simulink subsystem "packs_temperatures_12"  (R2020b)
settings: Solver=VariableStepAuto  StartTime=0.0  StopTime=10.0  RelTol=1e-3
undefined symbols (not defined in the file): bufferSize, params_packs_temperatures_12, possible_ppms
libraries: cstblocks x12
settings Model: Creator=leop9  LastModifiedBy=Previ

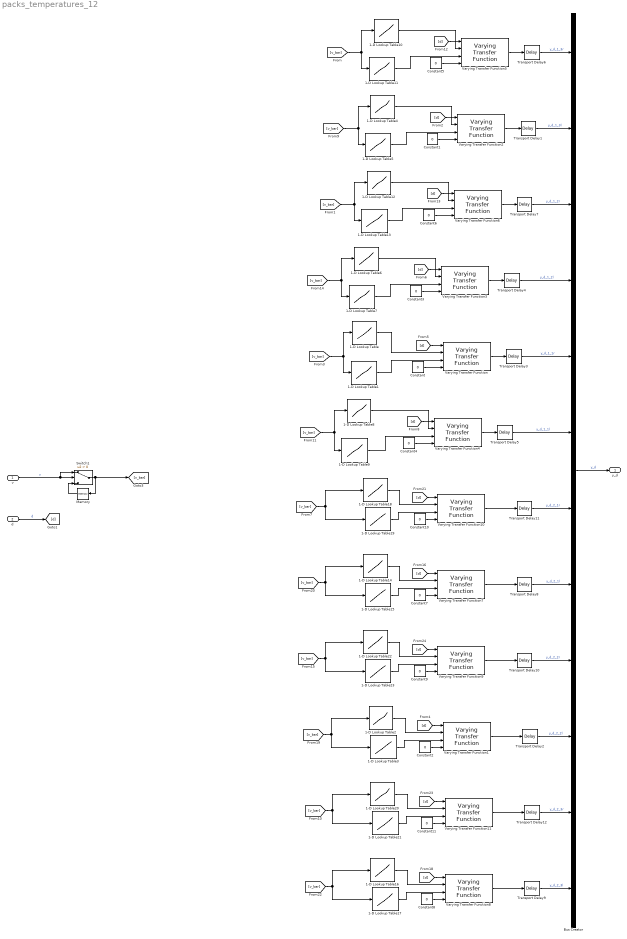
== system packs_temperatures_12 ==
  v : Inport
  d : Inport  Port=2
  1-D Lookup Table : Lookup_n-D  NumberOfTableDimensions=1  BreakpointsForDimension1=possible_ppms  BreakpointsForDimension2=[0,30,60,90]  Table=[params_packs_temperatures_12.T1_1r.b0(1),params_packs_temperatures_12.T1_1r.b0(2),params_packs_temperatures_12.T1_1r.b0(3)]  InternalRulePriority=Speed  RndMeth=Simplest  InputSameDT=on
  1-D Lookup Table1 : Lookup_n-D  NumberOfTableDimensions=1  BreakpointsForDimension1=possible_ppms  BreakpointsForDimension2=[0,30,60,90]  Table=[params_packs_temperatures_12.T1_1r.a0(1),params_packs_temperatures_12.T1_1r.a0(2),params_packs_temperatures_12.T1_1r.a0(3)]  InternalRulePriority=Speed  RndMeth=Simplest  InputSameDT=on
  1-D Lookup Table10 : Lookup_n-D  NumberOfTableDimensions=1  BreakpointsForDimension1=possible_ppms  BreakpointsForDimension2=[0,30,60,90]  Table=[params_packs_temperatures_12.T1_3r.b0(1),params_packs_temperatures_12.T1_3r.b0(2),params_packs_temperatures_12.T1_3r.b0(3)]  InternalRulePriority=Speed  RndMeth=Simplest  InputSameDT=on
  1-D Lookup Table11 : Lookup_n-D  NumberOfTableDimensions=1  BreakpointsForDimension1=possible_ppms  BreakpointsForDimension2=[0,30,60,90]  Table=[params_packs_temperatures_12.T1_3r.a0(1),params_packs_temperatures_12.T1_3r.a0(2),params_packs_temperatures_12.T1_3r.a0(3)]  InternalRulePriority=Speed  RndMeth=Simplest  InputSameDT=on
  1-D Lookup Table12 : Lookup_n-D  NumberOfTableDimensions=1  BreakpointsForDimension1=possible_ppms  BreakpointsForDimension2=[0,30,60,90]  Table=[params_packs_temperatures_12.T1_2r.b0(1),params_packs_temperatures_12.T1_2r.b0(2),params_packs_temperatures_12.T1_2r.b0(3)]  InternalRulePriority=Speed  RndMeth=Simplest  InputSameDT=on
  1-D Lookup Table13 : Lookup_n-D  NumberOfTableDimensions=1  BreakpointsForDimension1=possible_ppms  BreakpointsForDimension2=[0,30,60,90]  Table=[params_packs_temperatures_12.T1_2r.a0(1),params_packs_temperatures_12.T1_2r.a0(2),params_packs_temperatures_12.T1_2r.a0(3)]  InternalRulePriority=Speed  RndMeth=Simplest  InputSameDT=on
  1-D Lookup Table14 : Lookup_n-D  NumberOfTableDimensions=1  BreakpointsForDimension1=possible_ppms  BreakpointsForDimension2=[0,30,60,90]  Table=[params_packs_temperatures_12.T2_1l.b0(1),params_packs_temperatures_12.T2_1l.b0(2),params_packs_temperatures_12.T2_1l.b0(3)]  InternalRulePriority=Speed  RndMeth=Simplest  InputSameDT=on
  1-D Lookup Table15 : Lookup_n-D  NumberOfTableDimensions=1  BreakpointsForDimension1=possible_ppms  BreakpointsForDimension2=[0,30,60,90]  Table=[params_packs_temperatures_12.T2_1l.a0(1),params_packs_temperatures_12.T2_1l.a0(2),params_packs_temperatures_12.T2_1l.a0(3)]  InternalRulePriority=Speed  RndMeth=Simplest  InputSameDT=on
  1-D Lookup Table16 : Lookup_n-D  NumberOfTableDimensions=1  BreakpointsForDimension1=possible_ppms  BreakpointsForDimension2=[0,30,60,90]  Table=[params_packs_temperatures_12.T2_3l.b0(1),params_packs_temperatures_12.T2_3l.b0(2),params_packs_temperatures_12.T2_3l.b0(3)]  InternalRulePriority=Speed  RndMeth=Simplest  InputSameDT=on
  1-D Lookup Table17 : Lookup_n-D  NumberOfTableDimensions=1  BreakpointsForDimension1=possible_ppms  BreakpointsForDimension2=[0,30,60,90]  Table=[params_packs_temperatures_12.T2_3l.a0(1),params_packs_temperatures_12.T2_3l.a0(2),params_packs_temperatures_12.T2_3l.a0(3)]  InternalRulePriority=Speed  RndMeth=Simplest  InputSameDT=on
  1-D Lookup Table18 : Lookup_n-D  NumberOfTableDimensions=1  BreakpointsForDimension1=possible_ppms  BreakpointsForDimension2=[0,30,60,90]  Table=[params_packs_temperatures_12.T2_1r.b0(1),params_packs_temperatures_12.T2_1r.b0(2),params_packs_temperatures_12.T2_1r.b0(3)]  InternalRulePriority=Speed  RndMeth=Simplest  InputSameDT=on
  1-D Lookup Table19 : Lookup_n-D  NumberOfTableDimensions=1  BreakpointsForDimension1=possible_ppms  BreakpointsForDimension2=[0,30,60,90]  Table=[params_packs_temperatures_12.T2_1r.a0(1),params_packs_temperatures_12.T2_1r.a0(2),params_packs_temperatures_12.T2_1r.a0(3)]  InternalRulePriority=Speed  RndMeth=Simplest  InputSameDT=on
  1-D Lookup Table2 : Lookup_n-D  NumberOfTableDimensions=1  BreakpointsForDimension1=possible_ppms  BreakpointsForDimension2=[0,30,60,90]  Table=[params_packs_temperatures_12.T2_2l.b0(1),params_packs_temperatures_12.T2_2l.b0(2),params_packs_temperatures_12.T2_2l.b0(3)]  InternalRulePriority=Speed  RndMeth=Simplest  InputSameDT=on
  1-D Lookup Table20 : Lookup_n-D  NumberOfTableDimensions=1  BreakpointsForDimension1=possible_ppms  BreakpointsForDimension2=[0,30,60,90]  Table=[params_packs_temperatures_12.T2_3r.b0(1),params_packs_temperatures_12.T2_3r.b0(2),params_packs_temperatures_12.T2_3r.b0(3)]  InternalRulePriority=Speed  RndMeth=Simplest  InputSameDT=on
  1-D Lookup Table21 : Lookup_n-D  NumberOfTableDimensions=1  BreakpointsForDimension1=possible_ppms  BreakpointsForDimension2=[0,30,60,90]  Table=[params_packs_temperatures_12.T2_3r.a0(1),params_packs_temperatures_12.T2_3r.a0(2),params_packs_temperatures_12.T2_3r.a0(3)]  InternalRulePriority=Speed  RndMeth=Simplest  InputSameDT=on
  1-D Lookup Table22 : Lookup_n-D  NumberOfTableDimensions=1  BreakpointsForDimension1=possible_ppms  BreakpointsForDimension2=[0,30,60,90]  Table=[params_packs_temperatures_12.T2_2r.b0(1),params_packs_temperatures_12.T2_2r.b0(2),params_packs_temperatures_12.T2_2r.b0(3)]  InternalRulePriority=Speed  RndMeth=Simplest  InputSameDT=on
  1-D Lookup Table23 : Lookup_n-D  NumberOfTableDimensions=1  BreakpointsForDimension1=possible_ppms  BreakpointsForDimension2=[0,30,60,90]  Table=[params_packs_temperatures_12.T2_2r.a0(1),params_packs_temperatures_12.T2_2r.a0(2),params_packs_temperatures_12.T2_2r.a0(3)]  InternalRulePriority=Speed  RndMeth=Simplest  InputSameDT=on
  1-D Lookup Table3 : Lookup_n-D  NumberOfTableDimensions=1  BreakpointsForDimension1=possible_ppms  BreakpointsForDimension2=[0,30,60,90]  Table=[params_packs_temperatures_12.T2_2l.a0(1),params_packs_temperatures_12.T2_2l.a0(2),params_packs_temperatures_12.T2_2l.a0(3)]  InternalRulePriority=Speed  RndMeth=Simplest  InputSameDT=on
  1-D Lookup Table4 : Lookup_n-D  NumberOfTableDimensions=1  BreakpointsForDimension1=possible_ppms  BreakpointsForDimension2=[0,30,60,90]  Table=[params_packs_temperatures_12.T1_3l.b0(1),params_packs_temperatures_12.T1_3l.b0(2),params_packs_temperatures_12.T1_3l.b0(3)]  InternalRulePriority=Speed  RndMeth=Simplest  InputSameDT=on
  1-D Lookup Table5 : Lookup_n-D  NumberOfTableDimensions=1  BreakpointsForDimension1=possible_ppms  BreakpointsForDimension2=[0,30,60,90]  Table=[params_packs_temperatures_12.T1_3l.a0(1),params_packs_temperatures_12.T1_3l.a0(2),params_packs_temperatures_12.T1_3l.a0(3)]  InternalRulePriority=Speed  RndMeth=Simplest  InputSameDT=on
  1-D Lookup Table6 : Lookup_n-D  NumberOfTableDimensions=1  BreakpointsForDimension1=possible_ppms  BreakpointsForDimension2=[0,30,60,90]  Table=[params_packs_temperatures_12.T1_2l.b0(1),params_packs_temperatures_12.T1_2l.b0(2),params_packs_temperatures_12.T1_2l.b0(3)]  InternalRulePriority=Speed  RndMeth=Simplest  InputSameDT=on
  1-D Lookup Table7 : Lookup_n-D  NumberOfTableDimensions=1  BreakpointsForDimension1=possible_ppms  BreakpointsForDimension2=[0,30,60,90]  Table=[params_packs_temperatures_12.T1_2l.a0(1),params_packs_temperatures_12.T1_2l.a0(2),params_packs_temperatures_12.T1_2l.a0(3)]  InternalRulePriority=Speed  RndMeth=Simplest  InputSameDT=on
  1-D Lookup Table8 : Lookup_n-D  NumberOfTableDimensions=1  BreakpointsForDimension1=possible_ppms  BreakpointsForDimension2=[0,30,60,90]  Table=[params_packs_temperatures_12.T1_1l.b0(1),params_packs_temperatures_12.T1_1l.b0(2),params_packs_temperatures_12.T1_1l.b0(3)]  InternalRulePriority=Speed  RndMeth=Simplest  InputSameDT=on
  1-D Lookup Table9 : Lookup_n-D  NumberOfTableDimensions=1  BreakpointsForDimension1=possible_ppms  BreakpointsForDimension2=[0,30,60,90]  Table=[params_packs_temperatures_12.T1_1l.a0(1),params_packs_temperatures_12.T1_1l.a0(2),params_packs_temperatures_12.T1_1l.a0(3)]  InternalRulePriority=Speed  RndMeth=Simplest  InputSameDT=on
  Bus Creator : BusCreator  Inputs=12
  Constant{,1..11} (12 alike) : Constant  Value=0
  Memory : Memory
  Switch1 : Switch  Criteria=u2 > Threshold
  Transport Delay{1,3..7} (6 alike) : TransportDelay  DelayTime=params_packs_temperatures_12.T1_1r.delay  BufferSize=bufferSize
  Transport Delay{2,8..12} (6 alike) : TransportDelay  DelayTime=params_packs_temperatures_12.T2_2l.delay  BufferSize=bufferSize
  Varying Transfer Function{,1..11} (12 alike) : cstblocks/Linear Parameter Varying/Varying Transfer Function  N=1
  y_d : Outport
  wires:
  [v_bar] -> 1-D Lookup Table1/1, 1-D Lookup Table/1
  [v_bar] -> 1-D Lookup Table3/1, 1-D Lookup Table2/1
  1-D Lookup Table2/1 -> Varying Transfer Function1/2
  1-D Lookup Table3/1 -> Varying Transfer Function1/3
  Varying Transfer Function/1 -> Transport Delay3/1
  [d] -> Varying Transfer Function/1
  Varying Transfer Function1/1 -> Transport Delay2/1
  Constant/1 -> Varying Transfer Function/4
  Constant2/1 -> Varying Transfer Function1/4
  [d] -> Varying Transfer Function1/1
  1-D Lookup Table/1 -> Varying Transfer Function/2
  1-D Lookup Table1/1 -> Varying Transfer Function/3
  [d] -> Varying Transfer Function2/1
  1-D Lookup Table4/1 -> Varying Transfer Function2/2
  1-D Lookup Table5/1 -> Varying Transfer Function2/3
  Constant1/1 -> Varying Transfer Function2/4
  Varying Transfer Function2/1 -> Transport Delay1/1
  [v_bar] -> 1-D Lookup Table5/1, 1-D Lookup Table4/1
  Transport Delay1/1 -> Bus Creator/2  "y_d_1_3l"
  [v_bar] -> 1-D Lookup Table7/1, 1-D Lookup Table6/1
  Constant3/1 -> Varying Transfer Function3/4
  Varying Transfer Function3/1 -> Transport Delay4/1
  1-D Lookup Table7/1 -> Varying Transfer Function3/3
  1-D Lookup Table6/1 -> Varying Transfer Function3/2
  Transport Delay4/1 -> Bus Creator/4  "y_d_1_2l"
  [d] -> Varying Transfer Function3/1
  1-D Lookup Table8/1 -> Varying Transfer Function4/2
  Transport Delay5/1 -> Bus Creator/6  "y_d_1_1l"
  Varying Transfer Function4/1 -> Transport Delay5/1
  Constant4/1 -> Varying Transfer Function4/4
  [d] -> Varying Transfer Function4/1
  [v_bar] -> 1-D Lookup Table9/1, 1-D Lookup Table8/1
  1-D Lookup Table9/1 -> Varying Transfer Function4/3
  [v_bar] -> 1-D Lookup Table11/1, 1-D Lookup Table10/1
  Constant5/1 -> Varying Transfer Function5/4
  Varying Transfer Function5/1 -> Transport Delay6/1
  1-D Lookup Table11/1 -> Varying Transfer Function5/3
  1-D Lookup Table10/1 -> Varying Transfer Function5/2
  Transport Delay6/1 -> Bus Creator/1  "y_d_1_3r"
  [d] -> Varying Transfer Function5/1
  [d] -> Varying Transfer Function6/1
  [v_bar] -> 1-D Lookup Table13/1, 1-D Lookup Table12/1
  Varying Transfer Function6/1 -> Transport Delay7/1
  Constant6/1 -> Varying Transfer Function6/4
  1-D Lookup Table13/1 -> Varying Transfer Function6/3
  Transport Delay7/1 -> Bus Creator/3  "y_d_1_2r"
  1-D Lookup Table12/1 -> Varying Transfer Function6/2
  Transport Delay3/1 -> Bus Creator/5  "y_d_1_1r"
  [d] -> Varying Transfer Function7/1
  Varying Transfer Function7/1 -> Transport Delay8/1
  1-D Lookup Table14/1 -> Varying Transfer Function7/2
  [v_bar] -> 1-D Lookup Table15/1, 1-D Lookup Table14/1
  1-D Lookup Table15/1 -> Varying Transfer Function7/3
  Constant7/1 -> Varying Transfer Function7/4
  Transport Delay8/1 -> Bus Creator/8  "y_d_2_1l"
  Transport Delay2/1 -> Bus Creator/10  "y_d_2_2l"
  Transport Delay9/1 -> Bus Creator/12  "y_d_2_3l"
  [d] -> Varying Transfer Function8/1
  Varying Transfer Function8/1 -> Transport Delay9/1
  1-D Lookup Table16/1 -> Varying Transfer Function8/2
  [v_bar] -> 1-D Lookup Table17/1, 1-D Lookup Table16/1
  1-D Lookup Table17/1 -> Varying Transfer Function8/3
  Constant8/1 -> Varying Transfer Function8/4
  Transport Delay11/1 -> Bus Creator/7  "y_d_2_1r"
  1-D Lookup Table19/1 -> Varying Transfer Function10/3
  Constant10/1 -> Varying Transfer Function10/4
  Varying Transfer Function10/1 -> Transport Delay11/1
  [v_bar] -> 1-D Lookup Table19/1, 1-D Lookup Table18/1
  1-D Lookup Table18/1 -> Varying Transfer Function10/2
  Varying Transfer Function9/1 -> Transport Delay10/1
  1-D Lookup Table21/1 -> Varying Transfer Function11/3
  Constant11/1 -> Varying Transfer Function11/4
  1-D Lookup Table20/1 -> Varying Transfer Function11/2
  Transport Delay10/1 -> Bus Creator/9  "y_d_2_2r"
  Varying Transfer Function11/1 -> Transport Delay12/1
  [d] -> Varying Transfer Function11/1
  [d] -> Varying Transfer Function9/1
  Transport Delay12/1 -> Bus Creator/11  "y_d_2_3r"
  1-D Lookup Table22/1 -> Varying Transfer Function9/2
  [v_bar] -> 1-D Lookup Table21/1, 1-D Lookup Table20/1
  [v_bar] -> 1-D Lookup Table23/1, 1-D Lookup Table22/1
  [d] -> Varying Transfer Function10/1
  1-D Lookup Table23/1 -> Varying Transfer Function9/3
  Constant9/1 -> Varying Transfer Function9/4
  Switch1/1 -> [v_bar], Memory/1
  Memory/1 -> Switch1/3
  d/1 -> [d]  "d"
  v/1 -> Switch1/1, Switch1/2  "v"
  Bus Creator/1 -> y_d/1  "y_d"
